simulink model "rateLimit"  (R2015a)
settings: Solver=ode45  StartTime=0.0  StopTime=10.0  RelTol=1e-3
libraries: simulink x1
settings Model: Creator=Teme  LastModifiedBy=Teme
settings RTWCC: Toolchain=Clang v3.1 | gmake (64-bit Mac)

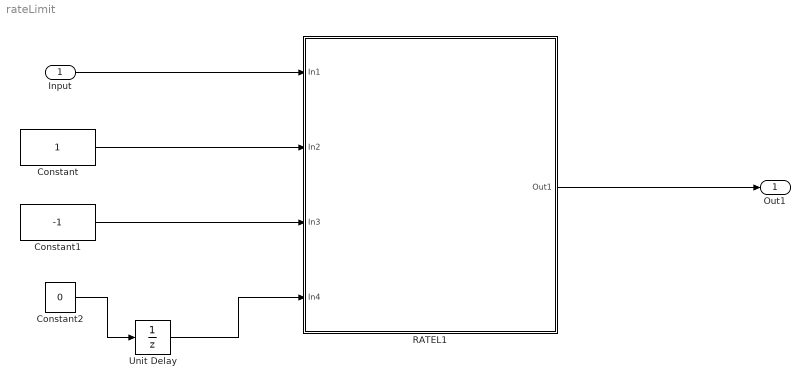
== system rateLimit ==
  Input : Inport
  Constant : Constant  OutDataTypeStr=single
  Constant1 : Constant  Value=-1  OutDataTypeStr=single
  Constant2 : Constant  Value=0  OutDataTypeStr=boolean
  RATEL1 : Subsystem  Description=Rate Limiter  mask{DT=0.01}
      mask prompts: DT "Input the Sample Time"
      settings: AttributesFormatString=%<Description>\nSample Time = %<DT>
      mask Display:
      | port_label('output', 1, 'Rate limited')
      | port_label('input', 1, 'Input')
      | port_label('input', 2, 'Rising Limit')
      | port_label('input', 3, 'Falling Limit')
      | port_label('input', 4, 'Init')
      | patch([0.35 .5 0.65], [0 .3 0], [0 1 0])
      | text(0.4,0.1, 'Safe')
  Unit Delay : UnitDelay  SampleTime=-1
  Out1 : Outport
  wires:
  Constant/1 -> RATEL1/2(In2)
  Constant1/1 -> RATEL1/3(In3)
  Constant2/1 -> Unit Delay/1
  RATEL1/1(Out1) -> Out1/1
  Unit Delay/1 -> RATEL1/4(In4)
  Input/1 -> RATEL1/1(In1)

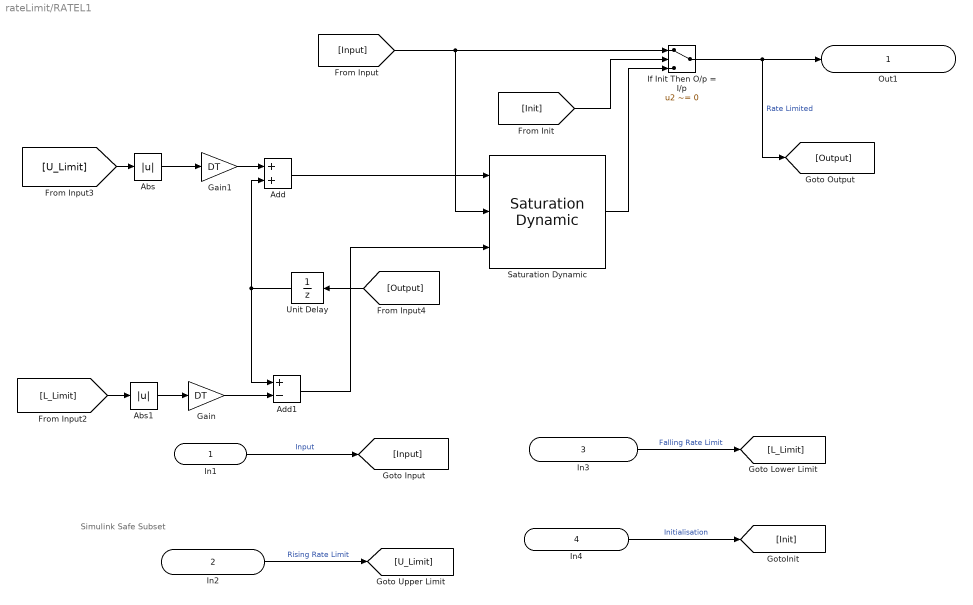
== system rateLimit/RATEL1 ==
  note: Simulink
      | Safe
      | Subset
  In1 : Inport  Description=Input Signal  OutDataTypeStr=single
      settings: AttributesFormatString=%<Description>\nPort No = %<Port>\nSample Time = %<SampleTime>\nSignal Type = %<SignalType>
  In2 : Inport  Description=Rising Limit  Port=2  OutDataTypeStr=single
      settings: AttributesFormatString=%<Description>\nPort No = %<Port>\nSample Time = %<SampleTime>\nSignal Type = %<SignalType>
  In3 : Inport  Description=Falling Limit  Port=3  OutDataTypeStr=single
      settings: AttributesFormatString=%<Description>\nPort No = %<Port>\nSample Time = %<SampleTime>\nSignal Type = %<SignalType>
  In4 : Inport  Description=Initialise  Port=4  OutDataTypeStr=boolean
      settings: AttributesFormatString=%<Description>\nPort No = %<Port>\nSample Time = %<SampleTime>\nSignal Type = %<SignalType>
  Abs : Abs
      settings: AttributesFormatString=ST = %<SampleTime>
  Abs1 : Abs
      settings: AttributesFormatString=ST = %<SampleTime>
  Add : Sum
      settings: AttributesFormatString=ST = %<SampleTime>
  Add1 : Sum  Inputs=+-
      settings: AttributesFormatString=ST = %<SampleTime>
  Gain : Gain  Gain=DT
  Gain1 : Gain  Gain=DT
  If Init Then O/p = I/p : Switch  Criteria=u2 ~= 0  Threshold=0.5  ZeroCross=off
      settings: AttributesFormatString=ST = %<SampleTime>\nThreshold = %<Threshold>\n%<Criteria>
  Saturation Dynamic : simulink/Discontinuities/Saturation Dynamic  OutMin=[]  OutMax=[]  OutDataTypeStr=Inherit: Same as second input  OutDataType=fixdt(1, 16)  OutScaling=2^-10  DoSatur=off
  Unit Delay : UnitDelay  SampleTime=-1
      settings: AttributesFormatString=ST = %<SampleTime>\nInitial = %<X0>
  Out1 : Outport  Description=Output Signal
      settings: AttributesFormatString=%<Description>\nPort No = %<Port>\nSample Time = %<SampleTime>\nSignal Type = %<SignalType>
  wires:
  Add1/1 -> Saturation Dynamic/3
  Add/1 -> Saturation Dynamic/1
  [Output] -> Unit Delay/1
  Gain1/1 -> Add/1
  [U_Limit] -> Abs/1
  Unit Delay/1 -> Add1/1, Add/2
  Gain/1 -> Add1/2
  [L_Limit] -> Abs1/1
  Saturation Dynamic/1 -> If Init Then O/p = I/p/3
  If Init Then O/p = I/p/1 -> [Output], Out1/1  "Rate Limited"
  [Init] -> If Init Then O/p = I/p/2
  In4/1 -> [Init]  "Initialisation"
  In3/1 -> [L_Limit]  "Falling Rate Limit"
  In2/1 -> [U_Limit]  "Rising Rate Limit"
  In1/1 -> [Input]  "Input"
  Abs/1 -> Gain1/1
  Abs1/1 -> Gain/1
  [Input] -> If Init Then O/p = I/p/1, Saturation Dynamic/2
